simulink model "DigitalTwin_v8"  (R2023a)
settings: Solver=ode23t  StartTime=0.0  StopTime=600  RelTol=1e-3  AbsTol=1e-3
model workspace: external: MATLAB File C:\Users\claud\OneDrive - TUM\COME -TUM\Software lab\Three_wheeled_base\simscape_1\Three_wheeled_base_DataFile1.m (data not in the file)
values from neighbouring files (symbols this model uses):
  brick_pick_global_xy = [brick_pick_global_xy, new_column]    [Three_wheeled_base_DataFile2.m]
  brick_place_global_xy = [brick_place_global_xy, new_column]    [Three_wheeled_base_DataFile2.m]
  platform_destination_mat = [ 1.0 0; 5 0; 0 0; 0 5 ... (first row only)    [Three_wheeled_base_DataFile2.m]
  robotData =     [points_on_pad.mat]
  smiData =     [points_on_pad.mat]    (also in road_points_on_pad.mat)
undefined symbols (not defined in the file or in its folder): X, Y, Z
libraries: sm_lib x246, nesl_utility x86, fl_lib x12, batteryecm_lib x5, ee_lib x3, robotcorelib x1, robotalgslib x1
(part 3 of 8)

== system DigitalTwin_v8/Subsystem1 ==
  Brick Position : Inport
  Theta Correction : Inport  Port=2
  Platform Position : Inport  Port=3
  Reshape1 : Reshape  OutputDimensionality=Customize  OutputDimensions=9
  Reshape2 : Reshape  OutputDimensionality=Customize  OutputDimensions=[3,3]
  Small delay : Subsystem
  Small delay1 : Subsystem
  Transfer Fcn3 : TransferFcn  Denominator=[10^(-6) 1]
  Out3 : Outport
  Out2 : Outport  Port=2
  platform_xy : Outport  Port=3
  wires:
  Platform Position/1 -> Small delay1/1(In1)
  Reshape1/1 -> Small delay/1(In1)
  Small delay/1(Out1) -> Reshape2/1
  Brick Position/1 -> Reshape1/1
  Reshape2/1 -> Out3/1
  Transfer Fcn3/1 -> Out2/1
  Theta Correction/1 -> Transfer Fcn3/1
  Small delay1/1(platform_xy) -> platform_xy/1

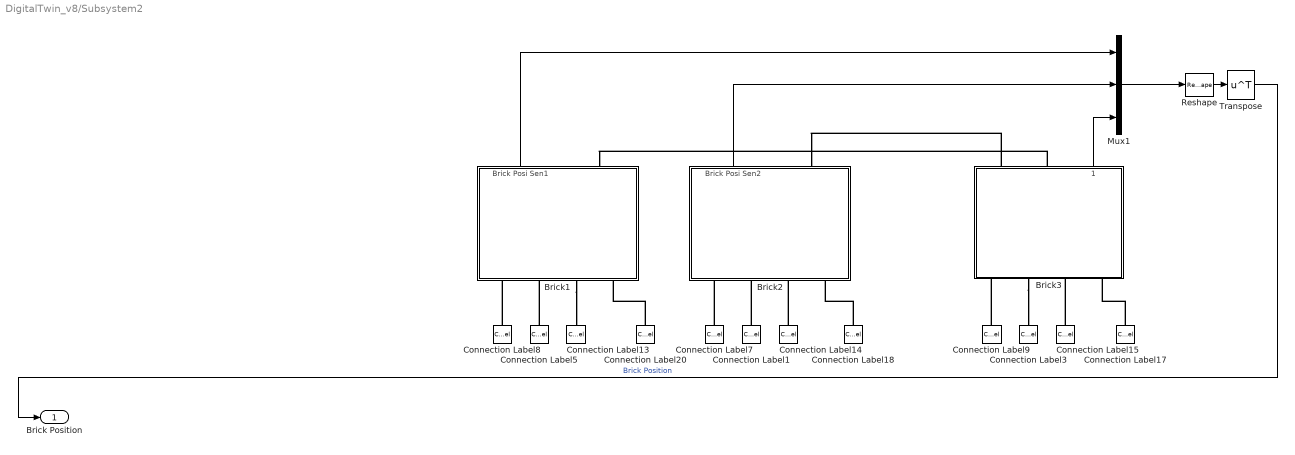
== system DigitalTwin_v8/Subsystem2 ==
  Brick1 : Subsystem
  Brick2 : Subsystem
  Brick3 : Subsystem
      settings: PortSchema="{\"entries\":[{\"content\":{\"sides\":[{\"content\":{\"connectorIds\":[\"LConn1\",\"LConn2\",\"LConn3\",\"LConn4\"]},\"type\":\"ConnectorPlacement.EquallySpacedRectSide\",\"uuid\":\"10c97bb1-3bf3-4133-85ed-799a328a8d18\"},{\"content\":{\"connectorIds\":[\"RConn1\",\"RConn2\",\"Out1\"],\"side\":\"RIGHT\"},\"type\":\"ConnectorPlacement.EquallySpacedRectSide\",\"uuid\":\"febed144-a77e-4bab-97e8-1b373a0f86c9\"},{\"content\":{\"side\":\"TOP\"},\"type\":\"ConnectorPlacement.EquallySpacedRectSide\",\"uuid\":\"baedfca3-20b6-436c-979e-46e0975f9023\"}]},\"type\":\"ConnectorPlacement.EquallySpacedConnector\",\"uuid\":\"f7b8695c-94a6-4ad5-b6b9-af354d139814\"}],\"packageUris\":[\"http://schema.mathworks.com/mf0/Connector/R2020b\"],\"version\":\"1.0\"}"
  Connection Label1 : ConnectionLabel  Label=WJ2
  Connection Label13 : ConnectionLabel  Label=Base_Ref
  Connection Label14 : ConnectionLabel  Label=Base_Ref
  Connection Label15 : ConnectionLabel  Label=Base_Ref
  Connection Label17 : ConnectionLabel  Label=BG_Contact3
  Connection Label18 : ConnectionLabel  Label=BG_Contact2
  Connection Label20 : ConnectionLabel  Label=BG_Contact1
  Connection Label3 : ConnectionLabel  Label=WJ3
  Connection Label5 : ConnectionLabel  Label=WJ1
  Connection Label7 : ConnectionLabel  Label=World_Ref
  Connection Label8 : ConnectionLabel  Label=World_Ref
  Connection Label9 : ConnectionLabel  Label=World_Ref
  Mux1 : Mux  Inputs=3
  Reshape : Reshape  OutputDimensionality=Customize  OutputDimensions=[3,3]
  Transpose : Math  Operator=transpose
  Brick Position : Outport
  wires:
  Brick1/1(Brick Posi Sen1) -> Mux1/1
  Brick2/1(Brick Posi Sen2) -> Mux1/2
  Brick3/1(Brick Posi Sen3) -> Mux1/3
  Transpose/1 -> Brick Position/1  "Brick Position"
  Reshape/1 -> Transpose/1
  Mux1/1 -> Reshape/1
  connections:
  Connection Label7/LConn1 -- Brick2/LConn1
  Connection Label14/LConn1 -- Brick2/LConn3
  Brick3/RConn1 -- Brick2/RConn1
  Connection Label17/LConn1 -- Brick3/LConn4
  Brick3/RConn2 -- Brick1/RConn1
  Brick3/LConn2 -- Connection Label3/LConn1
  Connection Label8/LConn1 -- Brick1/LConn1
  Connection Label5/LConn1 -- Brick1/LConn2
  Connection Label20/LConn1 -- Brick1/LConn4
  Connection Label15/LConn1 -- Brick3/LConn3
  Connection Label9/LConn1 -- Brick3/LConn1
  Connection Label1/LConn1 -- Brick2/LConn2
  Connection Label18/LConn1 -- Brick2/LConn4
  Brick1/LConn3 -- Connection Label13/LConn1

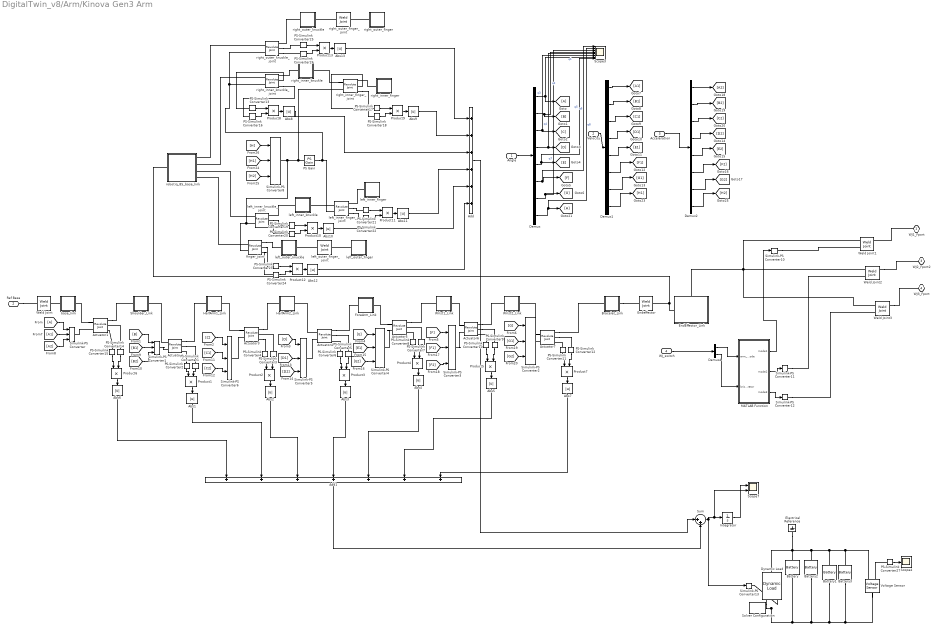
== system DigitalTwin_v8/Arm/Kinova Gen3 Arm ==
  Angle : Inport
  Velocity : Inport  Port=2
  Acceleration : Inport  Port=3
  WJ_switch : Inport  Port=4
  Abs{1..13} (13 alike) : Abs  ZeroCross=off  SaturateOnIntegerOverflow=off
  Actuator{1,3,5,7} (4 alike) : sm_lib/Joints/Revolute Joint  JointMode=Normal  SenseConstraintForce=off  SenseConstraintForceX=off  SenseConstraintForceY=off  SenseConstraintForceZ=off  SenseConstraintTorque=off  SenseConstraintTorqueX=off  SenseConstraintTorqueY=off  SenseConstraintTorqueZ=off  SenseTotalForce=off  SenseTotalForceX=off  SenseTotalForceY=off  SenseTotalForceZ=off  SenseTotalTorque=off  SenseTotalTorqueX=off  SenseTotalTorqueY=off  SenseTotalTorqueZ=off  CompositeWrenchDir=FollowerOnBase  CompositeWrenchFrame=BaseFrame  EquilibriumPosition=0  EquilibriumPositionUnits=deg  SpringStiffness=0  SpringStiffnessUnits=N*m/deg  DampingCoefficient=0.001  DampingCoefficientUnits=kg*m^2/(rad*s)  TorqueActuationMode=ComputedTorque  MotionActuationMode=InputMotion  SensePosition=off  SenseVelocity=on  SenseAcceleration=off  SenseTorqueForce=on  SenseLowerLimitTorqueForce=off  SenseUpperLimitTorqueForce=off  LowerLimitSpecify=off  LowerLimitBound=-90  LowerLimitBoundUnits=deg  LowerLimitStiffness=1e4  LowerLimitStiffnessUnits=N*m/deg  LowerLimitDamping=10  LowerLimitDampingUnits=N*m/(deg/s)  LowerLimitTransitionRegionWidth=0.1  LowerLimitTransitionRegionWidthUnits=deg  UpperLimitSpecify=off  UpperLimitBound=90  UpperLimitBoundUnits=deg  UpperLimitStiffness=1e4  UpperLimitStiffnessUnits=N*m/deg  UpperLimitDamping=10  UpperLimitDampingUnits=N*m/(deg/s)  UpperLimitTransitionRegionWidth=0.1  UpperLimitTransitionRegionWidthUnits=deg  PositionTargetSpecify=off  PositionTargetPriority=High  PositionTargetValue=0  PositionTargetValueUnits=deg  VelocityTargetSpecify=off  VelocityTargetPriority=High  VelocityTargetValue=0  VelocityTargetValueUnits=deg/s
  Actuator2 : sm_lib/Joints/Revolute Joint  JointMode=Normal  SenseConstraintForce=off  SenseConstraintForceX=off  SenseConstraintForceY=off  SenseConstraintForceZ=off  SenseConstraintTorque=off  SenseConstraintTorqueX=off  SenseConstraintTorqueY=off  SenseConstraintTorqueZ=off  SenseTotalForce=off  SenseTotalForceX=off  SenseTotalForceY=off  SenseTotalForceZ=off  SenseTotalTorque=off  SenseTotalTorqueX=off  SenseTotalTorqueY=off  SenseTotalTorqueZ=off  CompositeWrenchDir=FollowerOnBase  CompositeWrenchFrame=BaseFrame  EquilibriumPosition=0  EquilibriumPositionUnits=deg  SpringStiffness=0  SpringStiffnessUnits=N*m/deg  DampingCoefficient=0.001  DampingCoefficientUnits=kg*m^2/(rad*s)  TorqueActuationMode=ComputedTorque  MotionActuationMode=InputMotion  SensePosition=off  SenseVelocity=on  SenseAcceleration=off  SenseTorqueForce=on  SenseLowerLimitTorqueForce=off  SenseUpperLimitTorqueForce=off  LowerLimitSpecify=on  LowerLimitBound=-2.2  LowerLimitBoundUnits=rad  LowerLimitStiffness=1e4  LowerLimitStiffnessUnits=N*m/deg  LowerLimitDamping=10  LowerLimitDampingUnits=N*m/(deg/s)  LowerLimitTransitionRegionWidth=0.1  LowerLimitTransitionRegionWidthUnits=deg  UpperLimitSpecify=on  UpperLimitBound=2.2  UpperLimitBoundUnits=rad  UpperLimitStiffness=1e4  UpperLimitStiffnessUnits=N*m/deg  UpperLimitDamping=10  UpperLimitDampingUnits=N*m/(deg/s)  UpperLimitTransitionRegionWidth=0.1  UpperLimitTransitionRegionWidthUnits=deg  PositionTargetSpecify=off  PositionTargetPriority=High  PositionTargetValue=0  PositionTargetValueUnits=deg  VelocityTargetSpecify=off  VelocityTargetPriority=High  VelocityTargetValue=0  VelocityTargetValueUnits=deg/s
  Actuator4 : sm_lib/Joints/Revolute Joint  JointMode=Normal  SenseConstraintForce=off  SenseConstraintForceX=off  SenseConstraintForceY=off  SenseConstraintForceZ=off  SenseConstraintTorque=off  SenseConstraintTorqueX=off  SenseConstraintTorqueY=off  SenseConstraintTorqueZ=off  SenseTotalForce=off  SenseTotalForceX=off  SenseTotalForceY=off  SenseTotalForceZ=off  SenseTotalTorque=off  SenseTotalTorqueX=off  SenseTotalTorqueY=off  SenseTotalTorqueZ=off  CompositeWrenchDir=FollowerOnBase  CompositeWrenchFrame=BaseFrame  EquilibriumPosition=0  EquilibriumPositionUnits=deg  SpringStiffness=0  SpringStiffnessUnits=N*m/deg  DampingCoefficient=0.001  DampingCoefficientUnits=kg*m^2/(rad*s)  TorqueActuationMode=ComputedTorque  MotionActuationMode=InputMotion  SensePosition=off  SenseVelocity=on  SenseAcceleration=off  SenseTorqueForce=on  SenseLowerLimitTorqueForce=off  SenseUpperLimitTorqueForce=off  LowerLimitSpecify=on  LowerLimitBound=-2.5656  LowerLimitBoundUnits=rad  LowerLimitStiffness=1e4  LowerLimitStiffnessUnits=N*m/deg  LowerLimitDamping=10  LowerLimitDampingUnits=N*m/(deg/s)  LowerLimitTransitionRegionWidth=0.1  LowerLimitTransitionRegionWidthUnits=deg  UpperLimitSpecify=on  UpperLimitBound=2.5656  UpperLimitBoundUnits=rad  UpperLimitStiffness=1e4  UpperLimitStiffnessUnits=N*m/deg  UpperLimitDamping=10  UpperLimitDampingUnits=N*m/(deg/s)  UpperLimitTransitionRegionWidth=0.1  UpperLimitTransitionRegionWidthUnits=deg  PositionTargetSpecify=off  PositionTargetPriority=High  PositionTargetValue=0  PositionTargetValueUnits=deg  VelocityTargetSpecify=off  VelocityTargetPriority=High  VelocityTargetValue=0  VelocityTargetValueUnits=deg/s
  Actuator6 : sm_lib/Joints/Revolute Joint  JointMode=Normal  SenseConstraintForce=off  SenseConstraintForceX=off  SenseConstraintForceY=off  SenseConstraintForceZ=off  SenseConstraintTorque=off  SenseConstraintTorqueX=off  SenseConstraintTorqueY=off  SenseConstraintTorqueZ=off  SenseTotalForce=off  SenseTotalForceX=off  SenseTotalForceY=off  SenseTotalForceZ=off  SenseTotalTorque=off  SenseTotalTorqueX=off  SenseTotalTorqueY=off  SenseTotalTorqueZ=off  CompositeWrenchDir=FollowerOnBase  CompositeWrenchFrame=BaseFrame  EquilibriumPosition=0  EquilibriumPositionUnits=deg  SpringStiffness=0  SpringStiffnessUnits=N*m/deg  DampingCoefficient=0.001  DampingCoefficientUnits=kg*m^2/(rad*s)  TorqueActuationMode=ComputedTorque  MotionActuationMode=InputMotion  SensePosition=off  SenseVelocity=on  SenseAcceleration=off  SenseTorqueForce=on  SenseLowerLimitTorqueForce=off  SenseUpperLimitTorqueForce=off  LowerLimitSpecify=on  LowerLimitBound=-2.05  LowerLimitBoundUnits=rad  LowerLimitStiffness=1e4  LowerLimitStiffnessUnits=N*m/deg  LowerLimitDamping=10  LowerLimitDampingUnits=N*m/(deg/s)  LowerLimitTransitionRegionWidth=0.1  LowerLimitTransitionRegionWidthUnits=deg  UpperLimitSpecify=on  UpperLimitBound=2.05  UpperLimitBoundUnits=rad  UpperLimitStiffness=1e4  UpperLimitStiffnessUnits=N*m/deg  UpperLimitDamping=10  UpperLimitDampingUnits=N*m/(deg/s)  UpperLimitTransitionRegionWidth=0.1  UpperLimitTransitionRegionWidthUnits=deg  PositionTargetSpecify=off  PositionTargetPriority=High  PositionTargetValue=0  PositionTargetValueUnits=deg  VelocityTargetSpecify=off  VelocityTargetPriority=High  VelocityTargetValue=0  VelocityTargetValueUnits=deg/s
  Add : Sum  Inputs=++++++
  Add1 : Sum  Inputs=+++++++
  Battery{,1..3} (4 alike) : batteryecm_lib/Battery  Vnom=12 V  prm_dir=simscape.enum.battery.prm_dir.disabled  R1_dis=2 Ohm  R1_ch=2 Ohm  R1=2e-3 Ohm  prm_AH=simscape.enum.battery.prm_AH.infinite  AH=50 A*hr  V1=11.5 V  AH1=25 A*hr  prm_R2=simscape.enum.battery.prm_R2.disabled  R2=2000 Ohm  Tmeas=298.15 K  charge_measurement_port=simscape.enum.battery.enable.no  prm_dyn=simscape.enum.battery.prm_dyn.off  Rp1=0.005 Ohm  tau1=30 s  Rp2=0.005 Ohm  tau2=30 s  Rp3=0.005 Ohm  tau3=30 s  Rp4=0.005 Ohm  tau4=30 s  Rp5=0.005 Ohm  tau5=30 s  prm_fade=simscape.enum.battery.prm_fade.disabled  N_fade=100  AH_fade=45 A*hr  R1_fade=2.02 Ohm  R1_ch_fade=2.02 Ohm  V1_fade=10.35 V  prm_age=simscape.enum.battery.prm_age.disabled  prm_age_OCV=simscape.enum.battery.prm_age_OCV.OCV  OCV_age=0.9  SOC_age=60  Tmeas_age=298.15 K  delta_time_age_vec=[0] d  temperature_age_vec=[273] K  OCV_scaling_age=2.2134e6  OCV_offset_age=1.632e6  temp_exp_age=0.515833569 V  t_exp_age=0.75  Vnom_T2=12 V  R1_T2=2.2 Ohm  R1_T2_dis=2.2 Ohm  R1_T2_ch=2.2 Ohm  V1_T2=11.4 V  R2_T2=2200 Ohm  Rp1_T2=0.005 Ohm  tau1_T2=30 s  Rp2_T2=0.005 Ohm  tau2_T2=30 s  Rp3_T2=0.005 Ohm  tau3_T2=30 s  Rp4_T2=0.005 Ohm  tau4_T2=30 s  Rp5_T2=0.005 Ohm  tau5_T2=30 s  Tmeas2=273.15 K  thermal_port=simscape.enum.thermaleffects.omit  thermal_mass=30000 J/K  i_specify=off  i_priority=None  i=0 A  i_nominal_specify=off  i_nominal_unit=A  i_nominal_value=1  v_specify=off  v_priority=None  v=0 V  v_nominal_specify=off  v_nominal_unit=V  v_nominal_value=1  charge_specify=off  charge_priority=High  charge=50 A*hr  charge_nominal_specify=off  charge_nominal_unit=A*hr  charge_nominal_value=1  num_cycles_specify=off  num_cycles_priority=High  num_cycles=0  num_cycles_nominal_specify=off  num_cycles_nominal_unit=1  num_cycles_nominal_value=1  temperature_specify=off  temperature_priority=High  temperature=298.15 K  temperature_nominal_specify=off  temperature_nominal_unit=K  temperature_nominal_value=1
  Bracelet_Link : Subsystem
  Demux : Demux  Outputs=8
  Demux1 : Demux  Outputs=8
  Demux2 : Demux  Outputs=8
  Demux4 : Demux  Outputs=2
  Dynamic Load : ee_lib/Passive/Dynamic Load  load_type=ee.enum.dc_ac.dc  min_supply_voltage=20 V  pow_min=1e-3 W  G_reverse=1e-6 S  deltaV=1e-3 V  f0=60 Hz  Vrms_min=200 V  Pmin=1e-3 W  enable_fault=simscape.enum.onoff.off  fault_action=simscape.enum.assert.action.none  t_fault=1 s  open_conductance=1e-4 S
      settings: InternalSimscapePortConfiguration="{\"Bottom\":[],\"Left\":[{\"id\":\"p\",\"label\":\"+\",\"type\":\"foundation.electrical.electrical\"}],\"Right\":[{\"id\":\"n\",\"label\":\"-\",\"type\":\"foundation.electrical.electrical\"}],\"Top\":[{\"id\":\"P\",\"label\":\"P\",\"type\":\"input\"}]}"
  Electrical Reference : fl_lib/Electrical/Electrical Elements/Electrical Reference
  EndEffector_Link : Subsystem
      settings: PortSchema="{\"entries\":[{\"content\":{\"sides\":[{\"content\":{\"connectorIds\":[\"LConn1\"]},\"type\":\"ConnectorPlacement.EquallySpacedRectSide\",\"uuid\":\"82f16ba1-9569-4e63-828b-80ada8384267\"},{\"content\":{\"side\":\"RIGHT\"},\"type\":\"ConnectorPlacement.EquallySpacedRectSide\",\"uuid\":\"1c40a8b8-ff86-4403-bbc9-e3f7ed97d9c7\"},{\"content\":{\"connectorIds\":[\"LConn2\"],\"side\":\"TOP\"},\"type\":\"ConnectorPlacement.EquallySpacedRectSide\",\"uuid\":\"bd95f75a-cb9c-4683-98db-2a1a36a81fc6\"}]},\"type\":\"ConnectorPlacement.EquallySpacedConnector\",\"uuid\":\"3d9c398d-3d1c-44fe-8b52-b25795ae9eb8\"}],\"packageUris\":[\"http://schema.mathworks.com/mf0/Connector/R2020b\"],\"version\":\"1.0\"}"
  Endeffector : sm_lib/Joints/Weld Joint  JointMode=Normal  SenseConstraintForce=off  SenseConstraintForceX=off  SenseConstraintForceY=off  SenseConstraintForceZ=off  SenseConstraintTorque=off  SenseConstraintTorqueX=off  SenseConstraintTorqueY=off  SenseConstraintTorqueZ=off  SenseTotalForce=off  SenseTotalForceX=off  SenseTotalForceY=off  SenseTotalForceZ=off  SenseTotalTorque=off  SenseTotalTorqueX=off  SenseTotalTorqueY=off  SenseTotalTorqueZ=off  CompositeWrenchDir=FollowerOnBase  CompositeWrenchFrame=BaseFrame
  ForeArm_Link : Subsystem
  From : From
  Goto : Goto
  HalfArm1_Link : Subsystem
  HalfArm2_Link : Subsystem
  Integrator : Integrator
  MATLAB Function : MATLAB Function  TreatAsAtomicUnit=on
  PS Gain : fl_lib/Physical Signals/Functions/PS Gain  gain=-1
  PS-Simulink Converter{1..27} (27 alike) : nesl_utility/PS-Simulink Converter  PhysicalDomain=network_engine_domain  SubClassName=ps_output  LeftPortType=input  RightPortType=output  PseudoPeriodic=off  Frequencies=[]  VectorFormat=inherit  Unit=inherit  AffineConversion=off
  Product{1..13} (13 alike) : Product
  Scope3 : Scope  NumInputPorts=8
  Scope4 : Scope
  Scope7 : Scope  NumInputPorts=2
  Shoulder_Link : Subsystem
  Simulink-PS Converter{,1..6,8} (8 alike) : nesl_utility/Simulink-PS Converter  PhysicalDomain=network_engine_domain  SubClassName=ps_input  LeftPortType=input  RightPortType=output  PseudoPeriodic=off  Frequencies=[]  NoiseDistribution=none  NoiseParameters=[]  Unit=1  AffineConversion=off  FilteringAndDerivatives=provide  SimscapeFilterOrder=2  InputFilterTimeConstant=0.001  UdotUserProvided=2
  Simulink-PS Converter{10..13} (4 alike) : nesl_utility/Simulink-PS Converter  PhysicalDomain=network_engine_domain  SubClassName=ps_input  LeftPortType=input  RightPortType=output  PseudoPeriodic=off  Frequencies=[]  NoiseDistribution=none  NoiseParameters=[]  Unit=1  AffineConversion=off  FilteringAndDerivatives=provide  SimscapeFilterOrder=1  InputFilterTimeConstant=0.001  UdotUserProvided=0
  Solver Configuration : nesl_utility/Solver Configuration  PhysicalDomain=network_engine_domain  SubClassName=solver  LeftPortType=input  RightPortType=generic  Tones=[]  Harmonics=[]  SimulateNoise=off  Profile=off  UseLocalSampling=off  EnableSwitchedLinearOptims=on  FrequencyDomain=off  UseCCode=off  RelTol=0.001  AbsTol=0.001  MinStep=1e-09  ToWorkspace=off  RevertToSquareIcSolve=off  NumHomotopyIterations=100  PhasorMode=off  PhasorModeNumHarmonics=1  ConsistencySolver=NEWTON_XTOL_AFTER_FTOL  IndexReductionMethod=DerivativeReplacement  DoDC=off  ResidualTolerance=1e-09  ConsistencyTolSource=GLOBAL  ConsistencyAbsTol=0.001  ConsistencyRelTol=0.001  ConsistencyTolFactor=0.001  UseLocalSolver=off  LocalSolverChoice=NE_BACKWARD_EULER_ADVANCER  ResolveIndetEquations=on  FunctionEvalNumThread=1  LocalSolverSampleTime=0.001  DoFixedCost=off  MaxNonlinIter=3  MaxModeIter=2  ComputeImpulses=off  ImpulseIterations=2  LinearAlgebra=auto  LinearAlgebraNumThread=0  EquationFormulation=NE_TIME_EF  DelaysMemoryBudget=1024  AutomaticFiltering=on  FilteringTimeConstant=0.001  PartitionStorageMethod=AS_NEEDED  PartitionMemoryBudget=1024  PartitionMethod=ROBUST
  Sum : Sum  Inputs=|++
  Voltage Sensor : fl_lib/Electrical/Electrical Sensors/Voltage Sensor
  Weld Joint : sm_lib/Joints/Weld Joint  JointMode=Normal  SenseConstraintForce=off  SenseConstraintForceX=off  SenseConstraintForceY=off  SenseConstraintForceZ=off  SenseConstraintTorque=off  SenseConstraintTorqueX=off  SenseConstraintTorqueY=off  SenseConstraintTorqueZ=off  SenseTotalForce=off  SenseTotalForceX=off  SenseTotalForceY=off  SenseTotalForceZ=off  SenseTotalTorque=off  SenseTotalTorqueX=off  SenseTotalTorqueY=off  SenseTotalTorqueZ=off  CompositeWrenchDir=FollowerOnBase  CompositeWrenchFrame=BaseFrame
  Weld Joint1 : sm_lib/Joints/Weld Joint  JointMode=ProvidedByInput  SenseConstraintForce=off  SenseConstraintForceX=off  SenseConstraintForceY=off  SenseConstraintForceZ=off  SenseConstraintTorque=off  SenseConstraintTorqueX=off  SenseConstraintTorqueY=off  SenseConstraintTorqueZ=off  SenseTotalForce=on  SenseTotalForceX=off  SenseTotalForceY=off  SenseTotalForceZ=off  SenseTotalTorque=off  SenseTotalTorqueX=off  SenseTotalTorqueY=off  SenseTotalTorqueZ=off  CompositeWrenchDir=FollowerOnBase  CompositeWrenchFrame=BaseFrame
  Weld Joint2 : sm_lib/Joints/Weld Joint  JointMode=ProvidedByInput  SenseConstraintForce=off  SenseConstraintForceX=off  SenseConstraintForceY=off  SenseConstraintForceZ=off  SenseConstraintTorque=off  SenseConstraintTorqueX=off  SenseConstraintTorqueY=off  SenseConstraintTorqueZ=off  SenseTotalForce=on  SenseTotalForceX=off  SenseTotalForceY=off  SenseTotalForceZ=off  SenseTotalTorque=off  SenseTotalTorqueX=off  SenseTotalTorqueY=off  SenseTotalTorqueZ=off  CompositeWrenchDir=FollowerOnBase  CompositeWrenchFrame=BaseFrame
  Weld Joint3 : sm_lib/Joints/Weld Joint  JointMode=ProvidedByInput  SenseConstraintForce=off  SenseConstraintForceX=off  SenseConstraintForceY=off  SenseConstraintForceZ=off  SenseConstraintTorque=off  SenseConstraintTorqueX=off  SenseConstraintTorqueY=off  SenseConstraintTorqueZ=off  SenseTotalForce=on  SenseTotalForceX=off  SenseTotalForceY=off  SenseTotalForceZ=off  SenseTotalTorque=off  SenseTotalTorqueX=off  SenseTotalTorqueY=off  SenseTotalTorqueZ=off  CompositeWrenchDir=FollowerOnBase  CompositeWrenchFrame=BaseFrame
  Wrist1_Link : Subsystem
  Wrist2_Link : Subsystem
  base_link : Subsystem
  finger_joint : sm_lib/Joints/Revolute Joint  JointMode=Normal  SenseConstraintForce=off  SenseConstraintForceX=off  SenseConstraintForceY=off  SenseConstraintForceZ=off  SenseConstraintTorque=off  SenseConstraintTorqueX=off  SenseConstraintTorqueY=off  SenseConstraintTorqueZ=off  SenseTotalForce=off  SenseTotalForceX=off  SenseTotalForceY=off  SenseTotalForceZ=off  SenseTotalTorque=off  SenseTotalTorqueX=off  SenseTotalTorqueY=off  SenseTotalTorqueZ=off  CompositeWrenchDir=FollowerOnBase  CompositeWrenchFrame=BaseFrame  EquilibriumPosition=0  EquilibriumPositionUnits=deg  SpringStiffness=2  SpringStiffnessUnits=N*m/deg  DampingCoefficient=0.001  DampingCoefficientUnits=kg*m^2/(rad*s)  TorqueActuationMode=ComputedTorque  MotionActuationMode=InputMotion  SensePosition=off  SenseVelocity=on  SenseAcceleration=off  SenseTorqueForce=on  SenseLowerLimitTorqueForce=off  SenseUpperLimitTorqueForce=off  LowerLimitSpecify=on  LowerLimitBound=0  LowerLimitBoundUnits=rad  LowerLimitStiffness=1e4  LowerLimitStiffnessUnits=N*m/deg  LowerLimitDamping=10  LowerLimitDampingUnits=N*m/(deg/s)  LowerLimitTransitionRegionWidth=0.1  LowerLimitTransitionRegionWidthUnits=deg  UpperLimitSpecify=on  UpperLimitBound=0.725  UpperLimitBoundUnits=rad  UpperLimitStiffness=1e4  UpperLimitStiffnessUnits=N*m/deg  UpperLimitDamping=10  UpperLimitDampingUnits=N*m/(deg/s)  UpperLimitTransitionRegionWidth=0.1  UpperLimitTransitionRegionWidthUnits=deg  PositionTargetSpecify=off  PositionTargetPriority=High  PositionTargetValue=0  PositionTargetValueUnits=deg  VelocityTargetSpecify=off  VelocityTargetPriority=High  VelocityTargetValue=0  VelocityTargetValueUnits=deg/s
  left_inner_finger : Subsystem
  left_inner_finger_joint : sm_lib/Joints/Revolute Joint  JointMode=Normal  SenseConstraintForce=off  SenseConstraintForceX=off  SenseConstraintForceY=off  SenseConstraintForceZ=off  SenseConstraintTorque=off  SenseConstraintTorqueX=off  SenseConstraintTorqueY=off  SenseConstraintTorqueZ=off  SenseTotalForce=off  SenseTotalForceX=off  SenseTotalForceY=off  SenseTotalForceZ=off  SenseTotalTorque=off  SenseTotalTorqueX=off  SenseTotalTorqueY=off  SenseTotalTorqueZ=off  CompositeWrenchDir=FollowerOnBase  CompositeWrenchFrame=BaseFrame  EquilibriumPosition=0  EquilibriumPositionUnits=deg  SpringStiffness=2  SpringStiffnessUnits=N*m/deg  DampingCoefficient=0.001  DampingCoefficientUnits=kg*m^2/(rad*s)  TorqueActuationMode=ComputedTorque  MotionActuationMode=InputMotion  SensePosition=off  SenseVelocity=on  SenseAcceleration=off  SenseTorqueForce=on  SenseLowerLimitTorqueForce=off  SenseUpperLimitTorqueForce=off  LowerLimitSpecify=on  LowerLimitBound=0  LowerLimitBoundUnits=rad  LowerLimitStiffness=1e4  LowerLimitStiffnessUnits=N*m/deg  LowerLimitDamping=10  LowerLimitDampingUnits=N*m/(deg/s)  LowerLimitTransitionRegionWidth=0.1  LowerLimitTransitionRegionWidthUnits=deg  UpperLimitSpecify=on  UpperLimitBound=0.8757  UpperLimitBoundUnits=rad  UpperLimitStiffness=1e4  UpperLimitStiffnessUnits=N*m/deg  UpperLimitDamping=10  UpperLimitDampingUnits=N*m/(deg/s)  UpperLimitTransitionRegionWidth=0.1  UpperLimitTransitionRegionWidthUnits=deg  PositionTargetSpecify=off  PositionTargetPriority=High  PositionTargetValue=0  PositionTargetValueUnits=deg  VelocityTargetSpecify=off  VelocityTargetPriority=High  VelocityTargetValue=0  VelocityTargetValueUnits=deg/s
  left_inner_knuckle : Subsystem
  left_inner_knuckle_joint : sm_lib/Joints/Revolute Joint  JointMode=Normal  SenseConstraintForce=off  SenseConstraintForceX=off  SenseConstraintForceY=off  SenseConstraintForceZ=off  SenseConstraintTorque=off  SenseConstraintTorqueX=off  SenseConstraintTorqueY=off  SenseConstraintTorqueZ=off  SenseTotalForce=off  SenseTotalForceX=off  SenseTotalForceY=off  SenseTotalForceZ=off  SenseTotalTorque=off  SenseTotalTorqueX=off  SenseTotalTorqueY=off  SenseTotalTorqueZ=off  CompositeWrenchDir=FollowerOnBase  CompositeWrenchFrame=BaseFrame  EquilibriumPosition=0  EquilibriumPositionUnits=deg  SpringStiffness=2  SpringStiffnessUnits=N*m/deg  DampingCoefficient=0.001  DampingCoefficientUnits=kg*m^2/(rad*s)  TorqueActuationMode=ComputedTorque  MotionActuationMode=InputMotion  SensePosition=off  SenseVelocity=on  SenseAcceleration=off  SenseTorqueForce=on  SenseLowerLimitTorqueForce=off  SenseUpperLimitTorqueForce=off  LowerLimitSpecify=on  LowerLimitBound=0  LowerLimitBoundUnits=rad  LowerLimitStiffness=1e4  LowerLimitStiffnessUnits=N*m/deg  LowerLimitDamping=10  LowerLimitDampingUnits=N*m/(deg/s)  LowerLimitTransitionRegionWidth=0.1  LowerLimitTransitionRegionWidthUnits=deg  UpperLimitSpecify=on  UpperLimitBound=0.8757  UpperLimitBoundUnits=rad  UpperLimitStiffness=1e4  UpperLimitStiffnessUnits=N*m/deg  UpperLimitDamping=10  UpperLimitDampingUnits=N*m/(deg/s)  UpperLimitTransitionRegionWidth=0.1  UpperLimitTransitionRegionWidthUnits=deg  PositionTargetSpecify=off  PositionTargetPriority=High  PositionTargetValue=0  PositionTargetValueUnits=deg  VelocityTargetSpecify=off  VelocityTargetPriority=High  VelocityTargetValue=0  VelocityTargetValueUnits=deg/s
  left_outer_finger : Subsystem
  left_outer_finger_joint : sm_lib/Joints/Weld Joint  JointMode=Normal  SenseConstraintForce=off  SenseConstraintForceX=off  SenseConstraintForceY=off  SenseConstraintForceZ=off  SenseConstraintTorque=off  SenseConstraintTorqueX=off  SenseConstraintTorqueY=off  SenseConstraintTorqueZ=off  SenseTotalForce=off  SenseTotalForceX=off  SenseTotalForceY=off  SenseTotalForceZ=off  SenseTotalTorque=off  SenseTotalTorqueX=off  SenseTotalTorqueY=off  SenseTotalTorqueZ=off  CompositeWrenchDir=FollowerOnBase  CompositeWrenchFrame=BaseFrame
  left_outer_knuckle : Subsystem
  right_inner_finger : Subsystem
      settings: PortSchema="{\"entries\":[{\"content\":{\"sides\":[{\"content\":{\"connectorIds\":[\"LConn1\"]},\"type\":\"ConnectorPlacement.EquallySpacedRectSide\",\"uuid\":\"71922e3f-f3da-4f8e-a431-634d7177fd7d\"},{\"content\":{\"connectorIds\":[\"RConn1\"],\"side\":\"RIGHT\"},\"type\":\"ConnectorPlacement.EquallySpacedRectSide\",\"uuid\":\"a8c57a92-683e-476b-a46a-d436dda9422c\"},{\"content\":{\"side\":\"TOP\"},\"type\":\"ConnectorPlacement.EquallySpacedRectSide\",\"uuid\":\"e4481355-2c2a-4a91-9db8-21bbf7ccf224\"},{\"content\":{\"connectorIds\":[\"RConn2\"],\"side\":\"BOTTOM\"},\"type\":\"ConnectorPlacement.EquallySpacedRectSide\",\"uuid\":\"8b87cebb-658a-4fb3-839a-4b1c93f01fda\"}]},\"type\":\"ConnectorPlacement.EquallySpacedConnector\",\"uuid\":\"6c946504-5ea5-4a0c-9fc6-a1151345cbc2\"}],\"packageUris\":[\"http://schema.mathworks.com/mf0/Connector/R2020b\"],\"version\":\"1.0\"}"
  right_inner_finger_joint : sm_lib/Joints/Revolute Joint  JointMode=Normal  SenseConstraintForce=off  SenseConstraintForceX=off  SenseConstraintForceY=off  SenseConstraintForceZ=off  SenseConstraintTorque=off  SenseConstraintTorqueX=off  SenseConstraintTorqueY=off  SenseConstraintTorqueZ=off  SenseTotalForce=off  SenseTotalForceX=off  SenseTotalForceY=off  SenseTotalForceZ=off  SenseTotalTorque=off  SenseTotalTorqueX=off  SenseTotalTorqueY=off  SenseTotalTorqueZ=off  CompositeWrenchDir=FollowerOnBase  CompositeWrenchFrame=BaseFrame  EquilibriumPosition=0  EquilibriumPositionUnits=deg  SpringStiffness=2  SpringStiffnessUnits=N*m/deg  DampingCoefficient=0.001  DampingCoefficientUnits=kg*m^2/(rad*s)  TorqueActuationMode=ComputedTorque  MotionActuationMode=InputMotion  SensePosition=off  SenseVelocity=on  SenseAcceleration=off  SenseTorqueForce=on  SenseLowerLimitTorqueForce=off  SenseUpperLimitTorqueForce=off  LowerLimitSpecify=on  LowerLimitBound=0  LowerLimitBoundUnits=rad  LowerLimitStiffness=1e4  LowerLimitStiffnessUnits=N*m/deg  LowerLimitDamping=10  LowerLimitDampingUnits=N*m/(deg/s)  LowerLimitTransitionRegionWidth=0.1  LowerLimitTransitionRegionWidthUnits=deg  UpperLimitSpecify=on  UpperLimitBound=0.8757  UpperLimitBoundUnits=rad  UpperLimitStiffness=1e4  UpperLimitStiffnessUnits=N*m/deg  UpperLimitDamping=10  UpperLimitDampingUnits=N*m/(deg/s)  UpperLimitTransitionRegionWidth=0.1  UpperLimitTransitionRegionWidthUnits=deg  PositionTargetSpecify=off  PositionTargetPriority=High  PositionTargetValue=0  PositionTargetValueUnits=deg  VelocityTargetSpecify=off  VelocityTargetPriority=High  VelocityTargetValue=0  VelocityTargetValueUnits=deg/s
  right_inner_knuckle : Subsystem
  right_inner_knuckle_joint : sm_lib/Joints/Revolute Joint  JointMode=Normal  SenseConstraintForce=off  SenseConstraintForceX=off  SenseConstraintForceY=off  SenseConstraintForceZ=off  SenseConstraintTorque=off  SenseConstraintTorqueX=off  SenseConstraintTorqueY=off  SenseConstraintTorqueZ=off  SenseTotalForce=off  SenseTotalForceX=off  SenseTotalForceY=off  SenseTotalForceZ=off  SenseTotalTorque=off  SenseTotalTorqueX=off  SenseTotalTorqueY=off  SenseTotalTorqueZ=off  CompositeWrenchDir=FollowerOnBase  CompositeWrenchFrame=BaseFrame  EquilibriumPosition=0  EquilibriumPositionUnits=deg  SpringStiffness=2  SpringStiffnessUnits=N*m/deg  DampingCoefficient=0.001  DampingCoefficientUnits=kg*m^2/(rad*s)  TorqueActuationMode=ComputedTorque  MotionActuationMode=InputMotion  SensePosition=off  SenseVelocity=on  SenseAcceleration=off  SenseTorqueForce=on  SenseLowerLimitTorqueForce=off  SenseUpperLimitTorqueForce=off  LowerLimitSpecify=on  LowerLimitBound=0  LowerLimitBoundUnits=rad  LowerLimitStiffness=1e4  LowerLimitStiffnessUnits=N*m/deg  LowerLimitDamping=10  LowerLimitDampingUnits=N*m/(deg/s)  LowerLimitTransitionRegionWidth=0.1  LowerLimitTransitionRegionWidthUnits=deg  UpperLimitSpecify=on  UpperLimitBound=0.8757  UpperLimitBoundUnits=rad  UpperLimitStiffness=1e4  UpperLimitStiffnessUnits=N*m/deg  UpperLimitDamping=10  UpperLimitDampingUnits=N*m/(deg/s)  UpperLimitTransitionRegionWidth=0.1  UpperLimitTransitionRegionWidthUnits=deg  PositionTargetSpecify=off  PositionTargetPriority=High  PositionTargetValue=0  PositionTargetValueUnits=deg  VelocityTargetSpecify=off  VelocityTargetPriority=High  VelocityTargetValue=0  VelocityTargetValueUnits=deg/s
  right_outer_finger : Subsystem
  right_outer_finger_joint : sm_lib/Joints/Weld Joint  JointMode=Normal  SenseConstraintForce=off  SenseConstraintForceX=off  SenseConstraintForceY=off  SenseConstraintForceZ=off  SenseConstraintTorque=off  SenseConstraintTorqueX=off  SenseConstraintTorqueY=off  SenseConstraintTorqueZ=off  SenseTotalForce=off  SenseTotalForceX=off  SenseTotalForceY=off  SenseTotalForceZ=off  SenseTotalTorque=off  SenseTotalTorqueX=off  SenseTotalTorqueY=off  SenseTotalTorqueZ=off  CompositeWrenchDir=FollowerOnBase  CompositeWrenchFrame=BaseFrame
  right_outer_knuckle : Subsystem
  right_outer_knuckle_joint : sm_lib/Joints/Revolute Joint  JointMode=Normal  SenseConstraintForce=off  SenseConstraintForceX=off  SenseConstraintForceY=off  SenseConstraintForceZ=off  SenseConstraintTorque=off  SenseConstraintTorqueX=off  SenseConstraintTorqueY=off  SenseConstraintTorqueZ=off  SenseTotalForce=off  SenseTotalForceX=off  SenseTotalForceY=off  SenseTotalForceZ=off  SenseTotalTorque=off  SenseTotalTorqueX=off  SenseTotalTorqueY=off  SenseTotalTorqueZ=off  CompositeWrenchDir=FollowerOnBase  CompositeWrenchFrame=BaseFrame  EquilibriumPosition=0  EquilibriumPositionUnits=deg  SpringStiffness=2  SpringStiffnessUnits=N*m/deg  DampingCoefficient=0.001  DampingCoefficientUnits=kg*m^2/(rad*s)  TorqueActuationMode=ComputedTorque  MotionActuationMode=InputMotion  SensePosition=off  SenseVelocity=on  SenseAcceleration=off  SenseTorqueForce=on  SenseLowerLimitTorqueForce=off  SenseUpperLimitTorqueForce=off  LowerLimitSpecify=on  LowerLimitBound=0  LowerLimitBoundUnits=rad  LowerLimitStiffness=1e4  LowerLimitStiffnessUnits=N*m/deg  LowerLimitDamping=10  LowerLimitDampingUnits=N*m/(deg/s)  LowerLimitTransitionRegionWidth=0.1  LowerLimitTransitionRegionWidthUnits=deg  UpperLimitSpecify=on  UpperLimitBound=0.8757  UpperLimitBoundUnits=rad  UpperLimitStiffness=1e4  UpperLimitStiffnessUnits=N*m/deg  UpperLimitDamping=10  UpperLimitDampingUnits=N*m/(deg/s)  UpperLimitTransitionRegionWidth=0.1  UpperLimitTransitionRegionWidthUnits=deg  PositionTargetSpecify=off  PositionTargetPriority=High  PositionTargetValue=0  PositionTargetValueUnits=deg  VelocityTargetSpecify=off  VelocityTargetPriority=High  VelocityTargetValue=0  VelocityTargetValueUnits=deg/s
  robotiq_85_base_link : Subsystem
  WJ1_Fport : PMIOPort  Side=Right
  Ref Base : PMIOPort  Port=2  Side=Left
  WJ2_Fport2 : PMIOPort  Port=3  Side=Right
  WJ3_Fport : PMIOPort  Port=4  Side=Right
  wires:
  [G] -> Simulink-PS Converter2/1
  [F] -> Simulink-PS Converter3/1
  [D] -> Simulink-PS Converter5/1
  [C] -> Simulink-PS Converter6/1
  From/1 -> Simulink-PS Converter/1
  Demux/1 -> Scope3/7, Goto/1  "q1"
  Demux/2 -> Scope3/4, [B]  "q2"
  [E] -> Simulink-PS Converter4/1
  Demux/3 -> [C], Scope3/6  "q3"
  Demux/4 -> Scope3/5, [D]  "q4"
  Demux/5 -> Scope3/8, [E]  "q5"
  Demux/6 -> Scope3/1, [F]  "q6"
  Demux/7 -> Scope3/3, [G]  "q7"
  Angle/1 -> Demux/1
  Demux1/3 -> [C1]
  Demux1/2 -> [B1]
  Demux1/7 -> [G1]
  Demux1/5 -> [E1]
  Demux1/6 -> [F1]
  Demux1/4 -> [D1]
  Demux1/1 -> [A1]
  Velocity/1 -> Demux1/1
  [A1] -> Simulink-PS Converter/2
  [A2] -> Simulink-PS Converter/3
  Demux2/1 -> [A2]
  Demux2/7 -> [G2]
  Demux2/3 -> [C2]
  Demux2/5 -> [E2]
  Demux2/6 -> [F2]
  Demux2/2 -> [B2]
  Demux2/4 -> [D2]
  Acceleration/1 -> Demux2/1
  [C1] -> Simulink-PS Converter6/2
  [C2] -> Simulink-PS Converter6/3
  [D2] -> Simulink-PS Converter5/3
  [D1] -> Simulink-PS Converter5/2
  [E1] -> Simulink-PS Converter4/2
  [E2] -> Simulink-PS Converter4/3
  [F1] -> Simulink-PS Converter3/2
  [F2] -> Simulink-PS Converter3/3
  [G2] -> Simulink-PS Converter2/3
  [G1] -> Simulink-PS Converter2/2
  Demux/8 -> Scope3/2, [H]  "q8"
  Demux1/8 -> [H1]
  Demux2/8 -> [H2]
  [H] -> Simulink-PS Converter8/1
  [H2] -> Simulink-PS Converter8/3
  [H1] -> Simulink-PS Converter8/2
  [B] -> Simulink-PS Converter1/1
  WJ_switch/1 -> Demux4/1
  Demux4/1 -> MATLAB Function/1(arm_mode)
  Demux4/2 -> MATLAB Function/2(brick_iterator)
  MATLAB Function/1(mode1) -> Simulink-PS Converter10/1
  MATLAB Function/2(mode2) -> Simulink-PS Converter11/1
  MATLAB Function/3(mode3) -> Simulink-PS Converter12/1
  [B1] -> Simulink-PS Converter1/2
  [B2] -> Simulink-PS Converter1/3
  Product6/1 -> Abs6/1
  PS-Simulink Converter14/1 -> Product6/2
  PS-Simulink Converter15/1 -> Product6/1
  Product1/1 -> Abs1/1
  PS-Simulink Converter1/1 -> Product1/2
  PS-Simulink Converter2/1 -> Product1/1
  Product2/1 -> Abs2/1
  PS-Simulink Converter3/1 -> Product2/2
  PS-Simulink Converter4/1 -> Product2/1
  Product3/1 -> Abs3/1
  PS-Simulink Converter5/1 -> Product3/2
  PS-Simulink Converter6/1 -> Product3/1
  Product4/1 -> Abs4/1
  PS-Simulink Converter7/1 -> Product4/2
  PS-Simulink Converter8/1 -> Product4/1
  Product5/1 -> Abs5/1
  PS-Simulink Converter9/1 -> Product5/2
  PS-Simulink Converter10/1 -> Product5/1
  PS-Simulink Converter11/1 -> Product7/1
  Product7/1 -> Abs7/1
  PS-Simulink Converter12/1 -> Product7/2
  PS-Simulink Converter13/1 -> Product8/1
  Product8/1 -> Abs8/1
  PS-Simulink Converter16/1 -> Product8/2
  Product9/1 -> Abs9/1
  PS-Simulink Converter18/1 -> Product9/2
  PS-Simulink Converter17/1 -> Product9/1
  Product10/1 -> Abs10/1
  PS-Simulink Converter20/1 -> Product10/2
  PS-Simulink Converter19/1 -> Product10/1
  Product11/1 -> Abs11/1
  PS-Simulink Converter22/1 -> Product11/2
  PS-Simulink Converter21/1 -> Product11/1
  Product12/1 -> Abs12/1
  PS-Simulink Converter24/1 -> Product12/2
  PS-Simulink Converter23/1 -> Product12/1
  Product13/1 -> Abs13/1
  PS-Simulink Converter26/1 -> Product13/2
  PS-Simulink Converter25/1 -> Product13/1
  Abs13/1 -> Add/1
  Abs8/1 -> Add/3
  Abs9/1 -> Add/2
  Abs11/1 -> Add/4
  Abs10/1 -> Add/5
  Abs12/1 -> Add/6
  Abs6/1 -> Add1/1
  Abs1/1 -> Add1/2
  Abs2/1 -> Add1/3
  Abs3/1 -> Add1/4
  Abs4/1 -> Add1/5
  Abs5/1 -> Add1/6
  Abs7/1 -> Add1/7
  Add1/1 -> Sum/2
  Add/1 -> Sum/1
  PS-Simulink Converter27/1 -> Scope4/1
  Sum/1 -> Scope7/2, Integrator/1, Simulink-PS Converter13/1
  Integrator/1 -> Scope7/1
  connections:
  Actuator7/LConn1 -- Wrist2_Link/RConn1
  Actuator1/RConn1 -- Shoulder_Link/LConn1
  Actuator4/LConn2 -- Simulink-PS Converter5/RConn1
  Actuator5/LConn2 -- Simulink-PS Converter4/RConn1
  Actuator3/LConn2 -- Simulink-PS Converter6/RConn1
  Actuator4/RConn1 -- ForeArm_Link/LConn1
  Simulink-PS Converter3/RConn1 -- Actuator6/LConn2
  Actuator2/LConn1 -- Shoulder_Link/RConn1
  Actuator6/RConn1 -- Wrist2_Link/LConn1
  Actuator7/RConn1 -- Bracelet_Link/LConn1
  Actuator3/LConn1 -- HalfArm1_Link/RConn1
  Actuator4/LConn1 -- HalfArm2_Link/RConn1
  EndEffector_Link/LConn1 -- robotiq_85_base_link/LConn1 -- Endeffector/RConn1
  Actuator1/LConn1 -- base_link/RConn1
  Actuator6/LConn1 -- Wrist1_Link/RConn1
  Bracelet_Link/RConn1 -- Endeffector/LConn1
  Actuator5/RConn1 -- Wrist1_Link/LConn1
  Actuator5/LConn1 -- ForeArm_Link/RConn1
  Actuator2/RConn1 -- HalfArm1_Link/LConn1
  Actuator3/RConn1 -- HalfArm2_Link/LConn1
  Actuator7/LConn2 -- Simulink-PS Converter2/RConn1
  right_outer_finger/LConn1 -- right_outer_finger_joint/RConn1
  right_inner_finger_joint/LConn1 -- right_inner_knuckle/RConn1
  left_inner_knuckle/LConn1 -- left_inner_knuckle_joint/RConn1
  left_outer_finger_joint/LConn1 -- left_outer_knuckle/RConn1
  left_outer_finger/LConn1 -- left_outer_finger_joint/RConn1
  right_inner_finger/LConn1 -- right_inner_finger_joint/RConn1
  right_outer_finger_joint/LConn1 -- right_outer_knuckle/RConn1
  finger_joint/LConn1 -- robotiq_85_base_link/RConn4
  left_inner_knuckle_joint/LConn1 -- robotiq_85_base_link/RConn3
  left_inner_finger/LConn1 -- left_inner_finger_joint/RConn1
  right_outer_knuckle_joint/LConn1 -- robotiq_85_base_link/RConn1
  right_inner_knuckle/LConn1 -- right_inner_knuckle_joint/RConn1
  right_inner_knuckle_joint/LConn1 -- robotiq_85_base_link/RConn2
  right_outer_knuckle/LConn1 -- right_outer_knuckle_joint/RConn1
  left_inner_finger_joint/LConn1 -- left_inner_knuckle/RConn1
  finger_joint/RConn1 -- left_outer_knuckle/LConn1
  PS Gain/RConn1 -- left_inner_finger_joint/LConn2 -- right_outer_knuckle_joint/LConn2 -- right_inner_knuckle_joint/LConn2
  right_inner_finger_joint/LConn2 -- finger_joint/LConn2 -- left_inner_knuckle_joint/LConn2 -- Simulink-PS Converter8/RConn1 -- PS Gain/LConn1
  base_link/LConn1 -- Weld Joint/RConn1
  Ref Base/RConn1 -- Weld Joint/LConn1
  WJ1_Fport/RConn1 -- Weld Joint1/RConn1
  Simulink-PS Converter/RConn1 -- Actuator1/LConn2
  Simulink-PS Converter1/RConn1 -- Actuator2/LConn2
  Simulink-PS Converter10/RConn1 -- Weld Joint1/LConn2
  Weld Joint1/LConn1 -- Weld Joint3/LConn1 -- Weld Joint2/LConn1 -- EndEffector_Link/LConn2
  Weld Joint2/RConn1 -- WJ2_Fport2/RConn1
  Simulink-PS Converter11/RConn1 -- Weld Joint2/LConn2
  PS-Simulink Converter15/LConn1 -- Actuator1/RConn3
  PS-Simulink Converter14/LConn1 -- Actuator1/RConn2
  PS-Simulink Converter2/LConn1 -- Actuator2/RConn3
  Actuator2/RConn2 -- PS-Simulink Converter1/LConn1
  Actuator3/RConn3 -- PS-Simulink Converter4/LConn1
  PS-Simulink Converter3/LConn1 -- Actuator3/RConn2
  PS-Simulink Converter6/LConn1 -- Actuator4/RConn3
  Actuator4/RConn2 -- PS-Simulink Converter5/LConn1
  PS-Simulink Converter8/LConn1 -- Actuator5/RConn3
  PS-Simulink Converter7/LConn1 -- Actuator5/RConn2
  PS-Simulink Converter10/LConn1 -- Actuator6/RConn3
  Actuator6/RConn2 -- PS-Simulink Converter9/LConn1
  PS-Simulink Converter11/LConn1 -- Actuator7/RConn3
  Actuator7/RConn2 -- PS-Simulink Converter12/LConn1
  right_inner_knuckle_joint/RConn3 -- PS-Simulink Converter16/LConn1
  right_inner_knuckle_joint/RConn2 -- PS-Simulink Converter13/LConn1
  right_inner_finger_joint/RConn2 -- PS-Simulink Converter17/LConn1
  right_inner_finger_joint/RConn3 -- PS-Simulink Converter18/LConn1
  left_inner_knuckle_joint/RConn2 -- PS-Simulink Converter19/LConn1
  left_inner_knuckle_joint/RConn3 -- PS-Simulink Converter20/LConn1
  left_inner_finger_joint/RConn2 -- PS-Simulink Converter21/LConn1
  left_inner_finger_joint/RConn3 -- PS-Simulink Converter22/LConn1
  finger_joint/RConn2 -- PS-Simulink Converter23/LConn1
  finger_joint/RConn3 -- PS-Simulink Converter24/LConn1
  right_outer_knuckle_joint/RConn2 -- PS-Simulink Converter25/LConn1
  right_outer_knuckle_joint/RConn3 -- PS-Simulink Converter26/LConn1
  Battery/RConn1 -- Dynamic Load/RConn1 -- Electrical Reference/LConn1 -- Battery2/RConn1 -- Battery1/RConn1 -- Battery3/RConn1 -- Voltage Sensor/RConn2
  Dynamic Load/LConn2 -- Simulink-PS Converter13/RConn1
  Voltage Sensor/LConn1 -- Battery1/LConn1 -- Battery2/LConn1 -- Solver Configuration/RConn1 -- Dynamic Load/LConn1 -- Battery/LConn1 -- Battery3/LConn1
  Voltage Sensor/RConn1 -- PS-Simulink Converter27/LConn1
  Weld Joint3/RConn1 -- WJ3_Fport/RConn1
  Simulink-PS Converter12/RConn1 -- Weld Joint3/LConn2

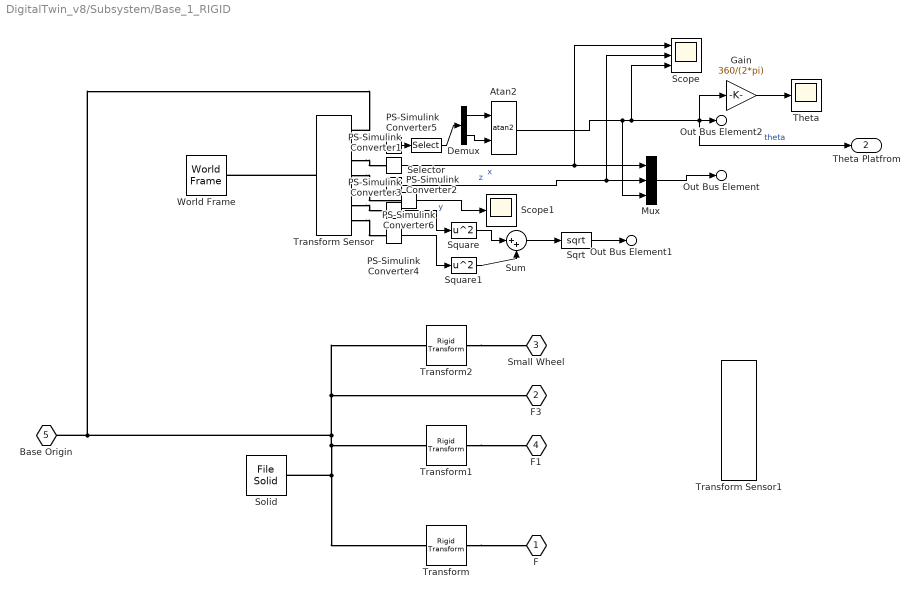
== system DigitalTwin_v8/Subsystem/Base_1_RIGID ==
  Atan2 : Trigonometry  Operator=atan2
  Demux : Demux  Outputs=2
  Gain : Gain  Gain=360/(2*pi)
  Mux : Mux  Inputs=3
  PS-Simulink Converter{1..6} (6 alike) : nesl_utility/PS-Simulink Converter  PhysicalDomain=network_engine_domain  SubClassName=ps_output  LeftPortType=input  RightPortType=output  PseudoPeriodic=off  Frequencies=[]  VectorFormat=inherit  Unit=inherit  AffineConversion=off
  Scope : Scope  NumInputPorts=3
  Scope1 : Scope
  Selector : Selector  NumberOfDimensions=2  InputPortWidth=3  IndexOptions=Index vector (dialog),Index vector (dialog)  Indices=[2,1],1  OutputSizes=1,1
  Solid : sm_lib/Body Elements/File Solid  ExtGeomFileName=Base_Predeterminado_sldprt.STEP  UnitType=FromFile  ExtGeomFileUnits=m  StepReaderType=HEX  ExportConvexHullGeometry=on  InertiaType=Custom  Mass=20  MassUnits=kg  CenterOfMass=smiData.Solid(5).CoM  CenterOfMassUnits=mm  MomentsOfInertia=smiData.Solid(5).MoI  MomentsOfInertiaUnits=kg*mm^2  ProductsOfInertia=smiData.Solid(5).PoI  ProductsOfInertiaUnits=kg*mm^2  BasedOnType=DensityFromFile  Density=1000  DensityUnits=kg/m^3  DoExposeReferenceFrame=on  SerializedFrames=<Frames/>  GraphicType=FromGeometry  MarkerShape=Sphere  MarkerSize=10  GraphicVisPropType=SimpleVisualProperties  GraphicDiffuseColor=smiData.Solid(5).color  GraphicSpecularColor=[0.5 0.5 0.5 1.0]  GraphicAmbientColor=[0.15 0.15 0.15 1.0]  GraphicEmissiveColor=[0.0 0.0 0.0 1.0]  GraphicShininess=75  GraphicOpacity=smiData.Solid(5).opacity
  Sqrt : Sqrt
  Square : Math  Operator=square
  Square1 : Math  Operator=square
  Sum : Sum  Inputs=|++
  Theta : Scope
  Transform : sm_lib/Frames and Transforms/Rigid Transform  TranslationMethod=Cartesian  TranslationStandardOffset=0  TranslationStandardOffsetUnits=m  TranslationStandardAxis=+Z  TranslationCartesianOffset=smiData.RigidTransform(1).translation  TranslationCartesianOffsetUnits=mm  TranslationROffset=0  TranslationROffsetUnits=m  TranslationZOffset=0  TranslationZOffsetUnits=m  TranslationThetaOffset=0  TranslationThetaOffsetUnits=deg  RotationMethod=ArbitraryAxis  RotationAngleUnits=rad  RotationStandardAxis=+Z  RotationAngle=smiData.RigidTransform(1).angle  RotationArbitraryAxis=smiData.RigidTransform(1).axis  FollAlignAxisA=+X  BaseAlignAxisA=+Y  FollAlignAxisB=+Y  BaseAlignAxisB=+Z  RotationSequenceAxes=FollowerAxes  RotationSequence=XYX  RotationSequenceAngles=[0 0 0]  RotationSequenceAnglesUnits=deg  RotationMatrix=[1 0 0; 0 1 0; 0 0 1]  Quaternion=[1 0 0 0]
  Transform Sensor : sm_lib/Frames and Transforms/Transform Sensor  MeasurementFrame=World  RotationSequence=XYX  SenseAngle=off  SenseAxis=off  SenseQ=off  SenseR=on  SenseRotationSequence=off  SenseOmegaX=off  SenseOmegaY=off  SenseOmegaZ=off  SenseQDot=off  SenseRDot=off  SenseRotationSequenceDot=off  SenseAlphaX=off  SenseAlphaY=off  SenseAlphaZ=off  SenseQDDot=off  SenseRDDot=off  SenseX=on  SenseY=on  SenseZ=on  SenseRad=off  SenseAzim=off  SenseDist=off  SenseInc=off  SenseXDot=on  SenseYDot=on  SenseZDot=off  SenseRadDot=off  SenseAzimDot=off  SenseDistDot=off  SenseIncDot=off  SenseXDDot=off  SenseYDDot=off  SenseZDDot=off  SenseRadDDot=off  SenseAzimDDot=off  SenseDistDDot=off  SenseIncDDot=off
  Transform Sensor1 : sm_lib/Frames and Transforms/Transform Sensor  MeasurementFrame=World  RotationSequence=XYX  SenseAngle=off  SenseAxis=off  SenseQ=off  SenseR=off  SenseRotationSequence=off  SenseOmegaX=off  SenseOmegaY=off  SenseOmegaZ=off  SenseQDot=off  SenseRDot=off  SenseRotationSequenceDot=off  SenseAlphaX=off  SenseAlphaY=off  SenseAlphaZ=off  SenseQDDot=off  SenseRDDot=off  SenseX=on  SenseY=on  SenseZ=off  SenseRad=off  SenseAzim=off  SenseDist=off  SenseInc=off  SenseXDot=on  SenseYDot=on  SenseZDot=off  SenseRadDot=off  SenseAzimDot=off  SenseDistDot=off  SenseIncDot=off  SenseXDDot=off  SenseYDDot=off  SenseZDDot=off  SenseRadDDot=off  SenseAzimDDot=off  SenseDistDDot=off  SenseIncDDot=off
  Transform1 : sm_lib/Frames and Transforms/Rigid Transform  TranslationMethod=Cartesian  TranslationStandardOffset=0  TranslationStandardOffsetUnits=m  TranslationStandardAxis=+Z  TranslationCartesianOffset=smiData.RigidTransform(3).translation  TranslationCartesianOffsetUnits=mm  TranslationROffset=0  TranslationROffsetUnits=m  TranslationZOffset=0  TranslationZOffsetUnits=m  TranslationThetaOffset=0  TranslationThetaOffsetUnits=deg  RotationMethod=ArbitraryAxis  RotationAngleUnits=rad  RotationStandardAxis=+Z  RotationAngle=smiData.RigidTransform(3).angle  RotationArbitraryAxis=smiData.RigidTransform(3).axis  FollAlignAxisA=+X  BaseAlignAxisA=+Y  FollAlignAxisB=+Y  BaseAlignAxisB=+Z  RotationSequenceAxes=FollowerAxes  RotationSequence=XYX  RotationSequenceAngles=[0 0 0]  RotationSequenceAnglesUnits=deg  RotationMatrix=[1 0 0; 0 1 0; 0 0 1]  Quaternion=[1 0 0 0]
  Transform2 : sm_lib/Frames and Transforms/Rigid Transform  TranslationMethod=Cartesian  TranslationStandardOffset=0  TranslationStandardOffsetUnits=m  TranslationStandardAxis=+Z  TranslationCartesianOffset=smiData.RigidTransform(5).translation  TranslationCartesianOffsetUnits=mm  TranslationROffset=0  TranslationROffsetUnits=m  TranslationZOffset=0  TranslationZOffsetUnits=m  TranslationThetaOffset=0  TranslationThetaOffsetUnits=deg  RotationMethod=ArbitraryAxis  RotationAngleUnits=rad  RotationStandardAxis=+Z  RotationAngle=smiData.RigidTransform(5).angle  RotationArbitraryAxis=smiData.RigidTransform(5).axis  FollAlignAxisA=+X  BaseAlignAxisA=+Y  FollAlignAxisB=+Y  BaseAlignAxisB=+Z  RotationSequenceAxes=FollowerAxes  RotationSequence=XYX  RotationSequenceAngles=[0 0 0]  RotationSequenceAnglesUnits=deg  RotationMatrix=[1 0 0; 0 1 0; 0 0 1]  Quaternion=[1 0 0 0]
  World Frame : sm_lib/Frames and Transforms/World Frame
  F : PMIOPort  Side=Left
  F3 : PMIOPort  Port=2  Side=Left
  Small Wheel : PMIOPort  Port=3  Side=Right
  F1 : PMIOPort  Port=4  Side=Right
  Base Origin : PMIOPort  Port=5  Side=Right
  Out Bus Element1 : Outport  PortName=Measure  Element=v
  Out Bus Element : Outport  PortName=Measure  Element=Position
  Out Bus Element2 : Outport  PortName=Measure  Element=theta
  Theta Platfrom : Outport  Port=2
  wires:
  PS-Simulink Converter1/1 -> Scope/1, Mux/1  "x"
  PS-Simulink Converter2/1 -> Scope/2, Mux/2  "z"
  Mux/1 -> Out Bus Element/1
  PS-Simulink Converter3/1 -> Square/1
  PS-Simulink Converter4/1 -> Square1/1
  Square/1 -> Sum/1
  Square1/1 -> Sum/2
  Sum/1 -> Sqrt/1
  Sqrt/1 -> Out Bus Element1/1
  PS-Simulink Converter5/1 -> Selector/1
  Demux/2 -> Atan2/2
  Demux/1 -> Atan2/1
  Selector/1 -> Demux/1
  Atan2/1 -> Theta Platfrom/1, Gain/1, Out Bus Element2/1, Scope/3, Mux/3  "theta"
  Gain/1 -> Theta/1
  PS-Simulink Converter6/1 -> Scope1/1  "y"
  connections:
  Transform/RConn1 -- F/RConn1
  Transform1/RConn1 -- F1/RConn1
  Transform2/RConn1 -- Small Wheel/RConn1
  Base Origin/RConn1 -- Transform2/LConn1 -- F3/RConn1 -- Solid/RConn1 -- Transform/LConn1 -- Transform1/LConn1 -- Transform Sensor/RConn1
  Transform Sensor/LConn1 -- World Frame/RConn1
  Transform Sensor/RConn2 -- PS-Simulink Converter5/LConn1
  Transform Sensor/RConn3 -- PS-Simulink Converter1/LConn1
  Transform Sensor/RConn4 -- PS-Simulink Converter2/LConn1
  Transform Sensor/RConn7 -- PS-Simulink Converter4/LConn1
  Transform Sensor/RConn6 -- PS-Simulink Converter3/LConn1
  Transform Sensor/RConn5 -- PS-Simulink Converter6/LConn1
